simulink model "LoFT_Example1"  (R2022b)
settings: Solver=ode4  StartTime=0.0  StopTime=500  FixedStep=simu.dt  RelTol=1e-3
PreLoadFcn:
  | simu.dt = 0.0125;
  | simu.Tmax = 600;
undefined symbols (not defined in the file): body, circtime, Communication, irkb, LoFT, Turbwind, waves, wind
libraries: simulink x25
(part 1 of 4)
settings Model: SimulationMode=accelerator  Creator=85164  LastModifiedBy=85164

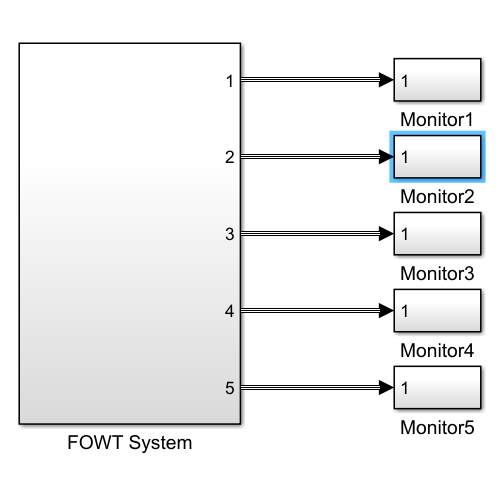
[thumbnail: Simulink's stored preview of the top-level diagram]
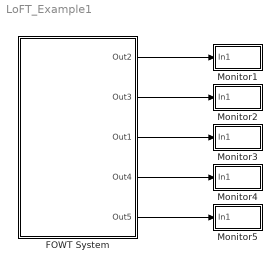
== system LoFT_Example1 ==
  FOWT System : Subsystem
  Monitor1 : Subsystem
  Monitor2 : Subsystem
  Monitor3 : Subsystem
  Monitor4 : Subsystem
  Monitor5 : Subsystem
  wires:
  FOWT System/1(Out2) -> Monitor1/1(In1)
  FOWT System/2(Out3) -> Monitor2/1(In1)
  FOWT System/3(Out1) -> Monitor3/1(In1)
  FOWT System/4(Out4) -> Monitor4/1(In1)
  FOWT System/5(Out5) -> Monitor5/1(In1)

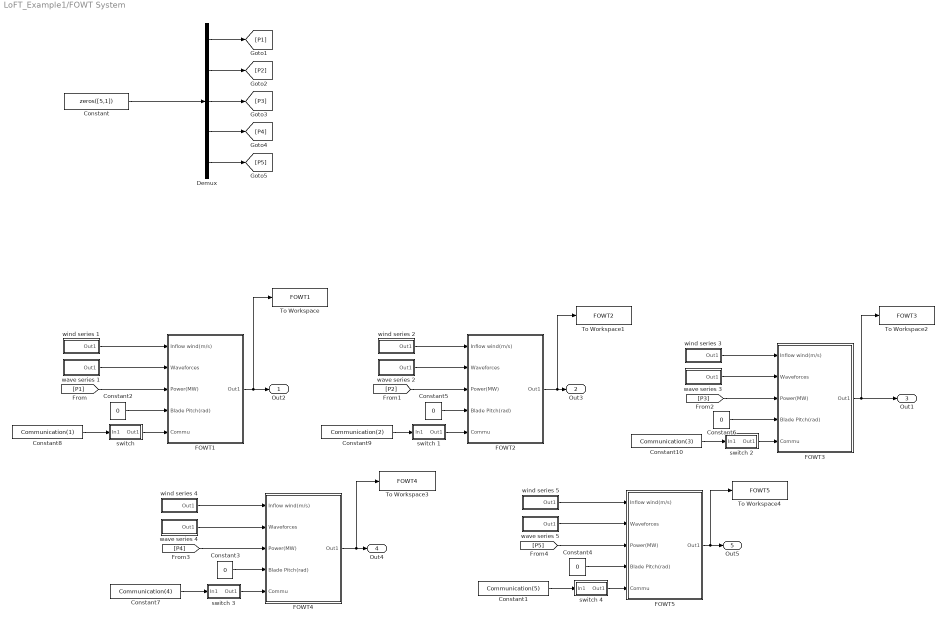
== system LoFT_Example1/FOWT System ==
  Constant : Constant  Value=zeros([5,1])
  Constant1 : Constant  Value=Communication(5)
  Constant10 : Constant  Value=Communication(3)
  Constant{2..6} (5 alike) : Constant  Value=0
  Constant7 : Constant  Value=Communication(4)
  Constant8 : Constant  Value=Communication(1)
  Constant9 : Constant  Value=Communication(2)
  Demux : Demux  Outputs=5
  FOWT1 : Subsystem  mask{Aero=LoFT.Aero, Hydro=LoFT.Hydro, Mooring=LoFT.Mooring, Property=LoFT.Property, Controller=LoFT.Controller, Initposition=[15,  0,  3*pi/180], Initstate=[6.8*pi/30, 9]}
      mask prompts: Aero "Aerodynamics"; Hydro "Hydrodynamics"; Mooring "Mooring lookup table"; Property "Hull mass, inertia and volume"; Controller "Local controller"; Initposition "Initial Hull position"; Initstate "Initial RotSpeed and WindEst"
      mask DialogControl DescGroupVar Prompt: LoFT
      mask DialogControl FOWT Prompt: Low-order modelling of floating offshore wind turbine for training
      mask DialogControl Manuscript Prompt: Citation
      mask DialogControl scriptname Prompt: Primary Frequency Response of Floating Offshore Wind Turbines via Deep Reinforcement Learning and Domain Randomization
      mask DialogControl ParameterGroupVar Prompt: 参数
  FOWT2 : Subsystem  mask{Aero=LoFT.Aero, Hydro=LoFT.Hydro, Mooring=LoFT.Mooring, Property=LoFT.Property, Controller=LoFT.Controller, Initposition=[15,  0,  3*pi/180], Initstate=[6.8*pi/30, 9]}
      mask prompts: Aero "Aerodynamics"; Hydro "Hydrodynamics"; Mooring "Mooring lookup table"; Property "Hull mass, inertia and volume"; Controller "Local controller"; Initposition "Initial Hull position"; Initstate "Initial RotSpeed and WindEst"
      mask DialogControl DescGroupVar Prompt: LoFT
      mask DialogControl FOWT Prompt: Low-order modelling of floating offshore wind turbine for training
      mask DialogControl Manuscript Prompt: Citation
      mask DialogControl scriptname Prompt: Primary Frequency Response of Floating Offshore Wind Turbines via Deep Reinforcement Learning and Domain Randomization
      mask DialogControl ParameterGroupVar Prompt: 参数
  FOWT3 : Subsystem  mask{Aero=LoFT.Aero, Hydro=LoFT.Hydro, Mooring=LoFT.Mooring, Property=LoFT.Property, Controller=LoFT.Controller, Initposition=[15,  0,  3*pi/180], Initstate=[6.8*pi/30, 9]}
      mask prompts: Aero "Aerodynamics"; Hydro "Hydrodynamics"; Mooring "Mooring lookup table"; Property "Hull mass, inertia and volume"; Controller "Local controller"; Initposition "Initial Hull position"; Initstate "Initial RotSpeed and WindEst"
      mask DialogControl DescGroupVar Prompt: LoFT
      mask DialogControl FOWT Prompt: Low-order modelling of floating offshore wind turbine for training
      mask DialogControl Manuscript Prompt: Citation
      mask DialogControl scriptname Prompt: Primary Frequency Response of Floating Offshore Wind Turbines via Deep Reinforcement Learning and Domain Randomization
      mask DialogControl ParameterGroupVar Prompt: 参数
  FOWT4 : Subsystem  mask{Aero=LoFT.Aero, Hydro=LoFT.Hydro, Mooring=LoFT.Mooring, Property=LoFT.Property, Controller=LoFT.Controller, Initposition=[15,  0,  3*pi/180], Initstate=[6.8*pi/30, 9]}
      mask prompts: Aero "Aerodynamics"; Hydro "Hydrodynamics"; Mooring "Mooring lookup table"; Property "Hull mass, inertia and volume"; Controller "Local controller"; Initposition "Initial Hull position"; Initstate "Initial RotSpeed and WindEst"
      mask DialogControl DescGroupVar Prompt: LoFT
      mask DialogControl FOWT Prompt: Low-order modelling of floating offshore wind turbine for training
      mask DialogControl Manuscript Prompt: Citation
      mask DialogControl scriptname Prompt: Primary Frequency Response of Floating Offshore Wind Turbines via Deep Reinforcement Learning and Domain Randomization
      mask DialogControl ParameterGroupVar Prompt: 参数
  FOWT5 : Subsystem  mask{Aero=LoFT.Aero, Hydro=LoFT.Hydro, Mooring=LoFT.Mooring, Property=LoFT.Property, Controller=LoFT.Controller, Initposition=[15,  0,  3*pi/180], Initstate=[6.8*pi/30, 9]}
      mask prompts: Aero "Aerodynamics"; Hydro "Hydrodynamics"; Mooring "Mooring lookup table"; Property "Hull mass, inertia and volume"; Controller "Local controller"; Initposition "Initial Hull position"; Initstate "Initial RotSpeed and WindEst"
      mask DialogControl DescGroupVar Prompt: LoFT
      mask DialogControl FOWT Prompt: Low-order modelling of floating offshore wind turbine for training
      mask DialogControl Manuscript Prompt: Citation
      mask DialogControl scriptname Prompt: Primary Frequency Response of Floating Offshore Wind Turbines via Deep Reinforcement Learning and Domain Randomization
      mask DialogControl ParameterGroupVar Prompt: 参数
  To Workspace : ToWorkspace  VariableName=FOWT1  SaveFormat=Timeseries  SampleTime=-1
  To Workspace1 : ToWorkspace  VariableName=FOWT2  SaveFormat=Timeseries  SampleTime=-1
  To Workspace2 : ToWorkspace  VariableName=FOWT3  SaveFormat=Timeseries  SampleTime=-1
  To Workspace3 : ToWorkspace  VariableName=FOWT4  SaveFormat=Timeseries  SampleTime=-1
  To Workspace4 : ToWorkspace  VariableName=FOWT5  SaveFormat=Timeseries  SampleTime=-1
  "switch " : Subsystem
  switch 1 : Subsystem
  switch 2 : Subsystem
  switch 3 : Subsystem
  switch 4 : Subsystem
  wave series 1 : Subsystem
  wave series 2 : Subsystem
  wave series 3 : Subsystem
  wave series 4 : Subsystem
  wave series 5 : Subsystem
  wind series 1 : Subsystem
  wind series 2 : Subsystem
  wind series 3 : Subsystem
  wind series 4 : Subsystem
  wind series 5 : Subsystem
  Out2 : Outport
  Out3 : Outport  Port=2
  Out1 : Outport  Port=3
  Out4 : Outport  Port=4
  Out5 : Outport  Port=5
  wires:
  switch 3/1(Out1) -> FOWT4/5(Commu)
  switch 4/1(Out1) -> FOWT5/5(Commu)
  wave series 4/1(Out1) -> FOWT4/2(Waveforces)
  switch 1/1(Out1) -> FOWT2/5(Commu)
  wave series 1/1(Out1) -> FOWT1/2(Waveforces)
  wave series 5/1(Out1) -> FOWT5/2(Waveforces)
  wave series 3/1(Out1) -> FOWT3/2(Waveforces)
  FOWT3/1(Out1) -> To Workspace2/1, Out1/1
  wave series 2/1(Out1) -> FOWT2/2(Waveforces)
  "switch "/1(Out1) -> FOWT1/5(Commu)
  switch 2/1(Out1) -> FOWT3/5(Commu)
  [P1] -> FOWT1/3(Power(MW))
  Constant2/1 -> FOWT1/4(Blade Pitch(rad))
  FOWT4/1(Out1) -> To Workspace3/1, Out4/1
  FOWT5/1(Out1) -> To Workspace4/1, Out5/1
  Constant1/1 -> switch 4/1(In1)
  [P2] -> FOWT2/3(Power(MW))
  [P3] -> FOWT3/3(Power(MW))
  Constant3/1 -> FOWT4/4(Blade Pitch(rad))
  Constant4/1 -> FOWT5/4(Blade Pitch(rad))
  Constant5/1 -> FOWT2/4(Blade Pitch(rad))
  Constant6/1 -> FOWT3/4(Blade Pitch(rad))
  Demux/1 -> [P1]
  Demux/5 -> [P5]
  Demux/4 -> [P4]
  Demux/3 -> [P3]
  Demux/2 -> [P2]
  [P4] -> FOWT4/3(Power(MW))
  [P5] -> FOWT5/3(Power(MW))
  FOWT2/1(Out1) -> To Workspace1/1, Out3/1
  Constant7/1 -> switch 3/1(In1)
  Constant8/1 -> "switch "/1(In1)
  Constant9/1 -> switch 1/1(In1)
  Constant10/1 -> switch 2/1(In1)
  Constant/1 -> Demux/1
  FOWT1/1(Out1) -> To Workspace/1, Out2/1
  wind series 5/1(Out1) -> FOWT5/1(Inflow wind(m/s))
  wind series 4/1(Out1) -> FOWT4/1(Inflow wind(m/s))
  wind series 3/1(Out1) -> FOWT3/1(Inflow wind(m/s))
  wind series 1/1(Out1) -> FOWT1/1(Inflow wind(m/s))
  wind series 2/1(Out1) -> FOWT2/1(Inflow wind(m/s))

== system LoFT_Example1/Monitor1 ==
  In1 : Inport
  Bus Selector : BusSelector  OutputSignals=PtfmSurge,PtfmHeave,PtfmPitch,WindVelX,WindEst,BldPitch,RotSpeed,GenPwr,RotThrust,GenTorq,RotTorq
  Gain : Gain  Gain=180/pi
  Gain1 : Gain  Gain=180/pi
  Scope : Scope  NumInputPorts=11
      settings: StartFcn=open_system(gcbh)
  wires:
  In1/1 -> Bus Selector/1
  Bus Selector/1 -> Scope/1  "<PtfmSurge>"
  Bus Selector/2 -> Scope/2  "<PtfmHeave>"
  Bus Selector/4 -> Scope/4  "<WindVelX>"
  Bus Selector/5 -> Scope/5  "<WindEst>"
  Bus Selector/7 -> Scope/7  "<RotSpeed>"
  Bus Selector/8 -> Scope/8  "<GenPwr>"
  Bus Selector/9 -> Scope/9  "<RotThrust>"
  Bus Selector/10 -> Scope/10  "<GenTorq>"
  Bus Selector/3 -> Gain/1  "<PtfmPitch>"
  Gain/1 -> Scope/3  "PtfmPitch"
  Bus Selector/6 -> Gain1/1  "<BldPitch>"
  Gain1/1 -> Scope/6  "BldPitch"
  Bus Selector/11 -> Scope/11  "<RotTorq>"

== system LoFT_Example1/Monitor2 ==
  In1 : Inport
  Bus Selector : BusSelector  OutputSignals=PtfmSurge,PtfmHeave,PtfmPitch,WindVelX,WindEst,BldPitch,RotSpeed,GenPwr,RotThrust,GenTorq,RotTorq
  Gain : Gain  Gain=180/pi
  Gain1 : Gain  Gain=180/pi
  Scope : Scope  NumInputPorts=11
  wires:
  Bus Selector/11 -> Scope/11  "<RotTorq>"
  Gain1/1 -> Scope/6  "BldPitch"
  Bus Selector/6 -> Gain1/1  "<BldPitch>"
  Gain/1 -> Scope/3  "PtfmPitch"
  Bus Selector/3 -> Gain/1  "<PtfmPitch>"
  Bus Selector/10 -> Scope/10  "<GenTorq>"
  Bus Selector/9 -> Scope/9  "<RotThrust>"
  Bus Selector/8 -> Scope/8  "<GenPwr>"
  Bus Selector/7 -> Scope/7  "<RotSpeed>"
  Bus Selector/5 -> Scope/5  "<WindEst>"
  Bus Selector/4 -> Scope/4  "<WindVelX>"
  Bus Selector/2 -> Scope/2  "<PtfmHeave>"
  Bus Selector/1 -> Scope/1  "<PtfmSurge>"
  In1/1 -> Bus Selector/1

== system LoFT_Example1/Monitor3 ==
  In1 : Inport
  Bus Selector : BusSelector  OutputSignals=PtfmSurge,PtfmHeave,PtfmPitch,WindVelX,WindEst,BldPitch,RotSpeed,GenPwr,RotThrust,GenTorq,RotTorq
  Gain : Gain  Gain=180/pi
  Gain1 : Gain  Gain=180/pi
  Scope : Scope  NumInputPorts=11
  wires:
  In1/1 -> Bus Selector/1
  Bus Selector/1 -> Scope/1  "<PtfmSurge>"
  Bus Selector/2 -> Scope/2  "<PtfmHeave>"
  Bus Selector/4 -> Scope/4  "<WindVelX>"
  Bus Selector/5 -> Scope/5  "<WindEst>"
  Bus Selector/7 -> Scope/7  "<RotSpeed>"
  Bus Selector/8 -> Scope/8  "<GenPwr>"
  Bus Selector/9 -> Scope/9  "<RotThrust>"
  Bus Selector/10 -> Scope/10  "<GenTorq>"
  Bus Selector/3 -> Gain/1  "<PtfmPitch>"
  Gain/1 -> Scope/3  "PtfmPitch"
  Bus Selector/6 -> Gain1/1  "<BldPitch>"
  Gain1/1 -> Scope/6  "BldPitch"
  Bus Selector/11 -> Scope/11  "<RotTorq>"

== system LoFT_Example1/Monitor4 ==
  In1 : Inport
  Bus Selector : BusSelector  OutputSignals=PtfmSurge,PtfmHeave,PtfmPitch,WindVelX,WindEst,BldPitch,RotSpeed,GenPwr,RotThrust,GenTorq,RotTorq
  Gain : Gain  Gain=180/pi
  Gain1 : Gain  Gain=180/pi
  Scope : Scope  NumInputPorts=11
  wires:
  Bus Selector/11 -> Scope/11  "<RotTorq>"
  Gain1/1 -> Scope/6  "BldPitch"
  Bus Selector/6 -> Gain1/1  "<BldPitch>"
  Gain/1 -> Scope/3  "PtfmPitch"
  Bus Selector/3 -> Gain/1  "<PtfmPitch>"
  Bus Selector/10 -> Scope/10  "<GenTorq>"
  Bus Selector/9 -> Scope/9  "<RotThrust>"
  Bus Selector/8 -> Scope/8  "<GenPwr>"
  Bus Selector/7 -> Scope/7  "<RotSpeed>"
  Bus Selector/5 -> Scope/5  "<WindEst>"
  Bus Selector/4 -> Scope/4  "<WindVelX>"
  Bus Selector/2 -> Scope/2  "<PtfmHeave>"
  Bus Selector/1 -> Scope/1  "<PtfmSurge>"
  In1/1 -> Bus Selector/1

== system LoFT_Example1/Monitor5 ==
  In1 : Inport
  Bus Selector : BusSelector  OutputSignals=PtfmSurge,PtfmHeave,PtfmPitch,WindVelX,WindEst,BldPitch,RotSpeed,GenPwr,RotThrust,GenTorq,RotTorq
  Gain : Gain  Gain=180/pi
  Gain1 : Gain  Gain=180/pi
  Scope : Scope  NumInputPorts=11
  wires:
  In1/1 -> Bus Selector/1
  Bus Selector/1 -> Scope/1  "<PtfmSurge>"
  Bus Selector/2 -> Scope/2  "<PtfmHeave>"
  Bus Selector/4 -> Scope/4  "<WindVelX>"
  Bus Selector/5 -> Scope/5  "<WindEst>"
  Bus Selector/7 -> Scope/7  "<RotSpeed>"
  Bus Selector/8 -> Scope/8  "<GenPwr>"
  Bus Selector/9 -> Scope/9  "<RotThrust>"
  Bus Selector/10 -> Scope/10  "<GenTorq>"
  Bus Selector/3 -> Gain/1  "<PtfmPitch>"
  Gain/1 -> Scope/3  "PtfmPitch"
  Bus Selector/6 -> Gain1/1  "<BldPitch>"
  Gain1/1 -> Scope/6  "BldPitch"
  Bus Selector/11 -> Scope/11  "<RotTorq>"

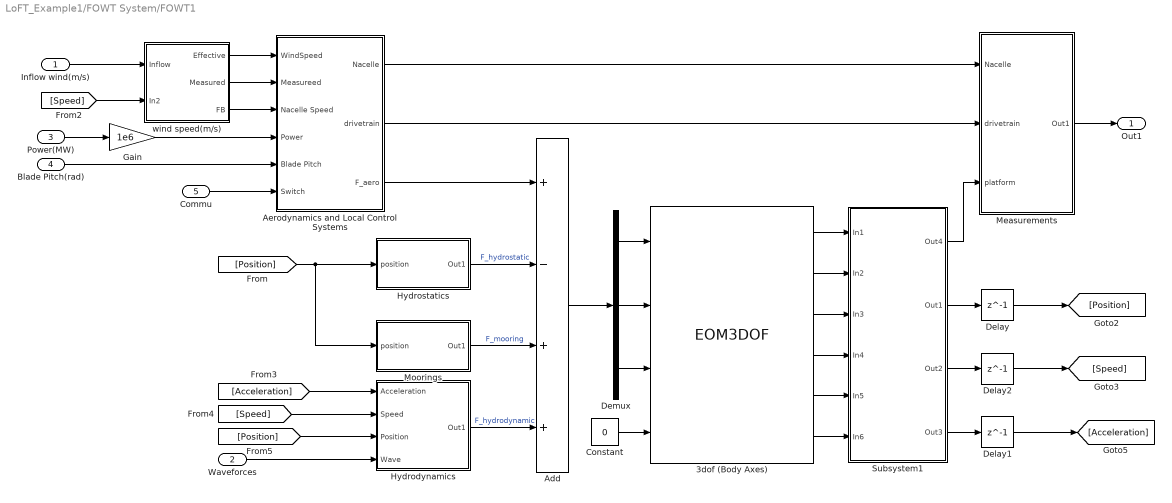
== system LoFT_Example1/FOWT System/FOWT1 ==
  Inflow wind(m/s) : Inport
  Waveforces : Inport  Port=2
  Power(MW) : Inport  Port=3
  Blade Pitch(rad) : Inport  Port=4
  Commu : Inport  Port=5
  3dof (Body Axes) : EOM3DOF  v_ini=0.01  theta_ini=Initposition(3)  pos_ini=[Initposition(1) Initposition(2)]  mass=Property.masstot  Iyy=Property.pitchinertia  g_in=External
  Add : Sum  Inputs=+-++
  Aerodynamics and Local Control Systems : Subsystem
  Constant : Constant  Value=0
  Delay : Delay  DelayLength=1  InitialCondition=0
  Delay1 : Delay  DelayLength=1  InitialCondition=0
  Delay2 : Delay  DelayLength=1  InitialCondition=0
  Demux : Demux  Outputs=3
  Gain : Gain  Gain=1e6
  Hydrodynamics : Subsystem
  Hydrostatics : Subsystem
  Measurements : Subsystem
  Moorings : Subsystem
  Subsystem1 : Subsystem
  wind speed(m/s) : Subsystem
  Out1 : Outport
  wires:
  Power(MW)/1 -> Gain/1
  wind speed(m/s)/3(FB) -> Aerodynamics and Local Control Systems/3(Nacelle Speed)
  Aerodynamics and Local Control Systems/2(drivetrain) -> Measurements/2(drivetrain)
  Measurements/1(Out1) -> Out1/1
  Aerodynamics and Local Control Systems/1(Nacelle) -> Measurements/1(Nacelle)
  Subsystem1/1(Out4) -> Measurements/3(platform)
  Waveforces/1 -> Hydrodynamics/4(Wave)
  Commu/1 -> Aerodynamics and Local Control Systems/6(Switch)
  Aerodynamics and Local Control Systems/3(F_aero) -> Add/1
  [Speed] -> wind speed(m/s)/2(In2)
  [Position] -> Hydrodynamics/3(Position)
  Hydrodynamics/1(Out1) -> Add/4  "F_hydrodynamic"
  [Speed] -> Hydrodynamics/2(Speed)
  Demux/3 -> 3dof (Body Axes)/3
  Demux/2 -> 3dof (Body Axes)/2
  Demux/1 -> 3dof (Body Axes)/1
  Add/1 -> Demux/1
  3dof (Body Axes)/6 -> Subsystem1/6(In6)
  3dof (Body Axes)/5 -> Subsystem1/5(In5)
  3dof (Body Axes)/4 -> Subsystem1/4(In4)
  3dof (Body Axes)/3 -> Subsystem1/3(In3)
  3dof (Body Axes)/2 -> Subsystem1/2(In2)
  3dof (Body Axes)/1 -> Subsystem1/1(In1)
  Moorings/1(Out1) -> Add/3  "F_mooring"
  Constant/1 -> 3dof (Body Axes)/4
  Hydrostatics/1(Out1) -> Add/2  "F_hydrostatic"
  [Position] -> Hydrostatics/1(position), Moorings/1(position)
  wind speed(m/s)/1(Effective) -> Aerodynamics and Local Control Systems/1(WindSpeed)
  Subsystem1/2(Out1) -> Delay/1
  Gain/1 -> Aerodynamics and Local Control Systems/4(Power)
  Subsystem1/3(Out2) -> Delay2/1
  Subsystem1/4(Out3) -> Delay1/1
  Inflow wind(m/s)/1 -> wind speed(m/s)/1(Inflow)
  Delay1/1 -> [Acceleration]
  Delay2/1 -> [Speed]
  Delay/1 -> [Position]
  [Acceleration] -> Hydrodynamics/1(Acceleration)
  wind speed(m/s)/2(Measured) -> Aerodynamics and Local Control Systems/2("Measureed ")
  Blade Pitch(rad)/1 -> Aerodynamics and Local Control Systems/5(Blade Pitch)

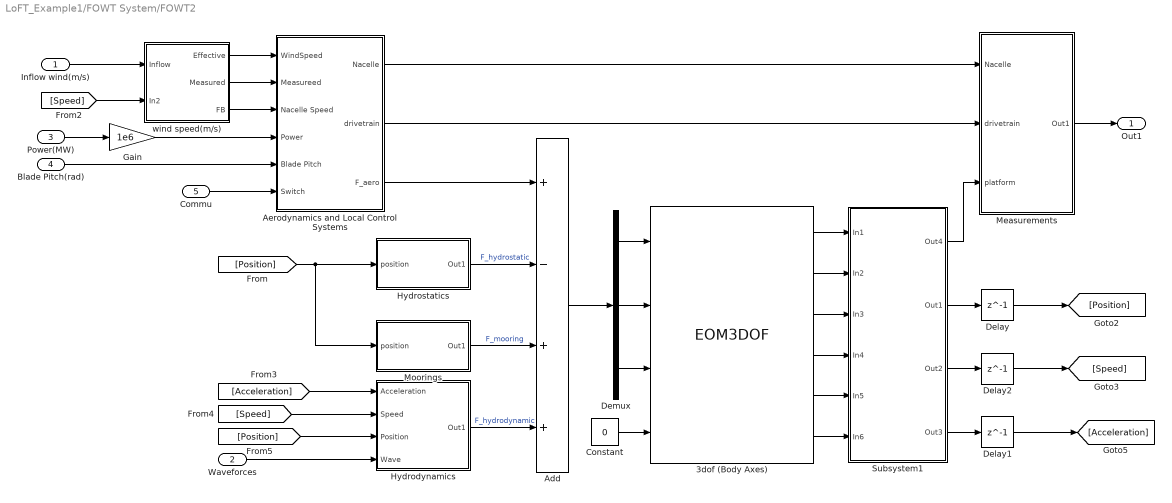
== system LoFT_Example1/FOWT System/FOWT2 ==
  Inflow wind(m/s) : Inport
  Waveforces : Inport  Port=2
  Power(MW) : Inport  Port=3
  Blade Pitch(rad) : Inport  Port=4
  Commu : Inport  Port=5
  3dof (Body Axes) : EOM3DOF  v_ini=0.01  theta_ini=Initposition(3)  pos_ini=[Initposition(1) Initposition(2)]  mass=Property.masstot  Iyy=Property.pitchinertia  g_in=External
  Add : Sum  Inputs=+-++
  Aerodynamics and Local Control Systems : Subsystem
  Constant : Constant  Value=0
  Delay : Delay  DelayLength=1  InitialCondition=0
  Delay1 : Delay  DelayLength=1  InitialCondition=0
  Delay2 : Delay  DelayLength=1  InitialCondition=0
  Demux : Demux  Outputs=3
  Gain : Gain  Gain=1e6
  Hydrodynamics : Subsystem
  Hydrostatics : Subsystem
  Measurements : Subsystem
  Moorings : Subsystem
  Subsystem1 : Subsystem
  wind speed(m/s) : Subsystem
  Out1 : Outport
  wires:
  Blade Pitch(rad)/1 -> Aerodynamics and Local Control Systems/5(Blade Pitch)
  wind speed(m/s)/2(Measured) -> Aerodynamics and Local Control Systems/2("Measureed ")
  [Acceleration] -> Hydrodynamics/1(Acceleration)
  Delay/1 -> [Position]
  Delay2/1 -> [Speed]
  Delay1/1 -> [Acceleration]
  Inflow wind(m/s)/1 -> wind speed(m/s)/1(Inflow)
  Subsystem1/4(Out3) -> Delay1/1
  Subsystem1/3(Out2) -> Delay2/1
  Gain/1 -> Aerodynamics and Local Control Systems/4(Power)
  Subsystem1/2(Out1) -> Delay/1
  wind speed(m/s)/1(Effective) -> Aerodynamics and Local Control Systems/1(WindSpeed)
  [Position] -> Moorings/1(position), Hydrostatics/1(position)
  Hydrostatics/1(Out1) -> Add/2  "F_hydrostatic"
  Constant/1 -> 3dof (Body Axes)/4
  Moorings/1(Out1) -> Add/3  "F_mooring"
  3dof (Body Axes)/1 -> Subsystem1/1(In1)
  3dof (Body Axes)/2 -> Subsystem1/2(In2)
  3dof (Body Axes)/3 -> Subsystem1/3(In3)
  3dof (Body Axes)/4 -> Subsystem1/4(In4)
  3dof (Body Axes)/5 -> Subsystem1/5(In5)
  3dof (Body Axes)/6 -> Subsystem1/6(In6)
  Add/1 -> Demux/1
  Demux/1 -> 3dof (Body Axes)/1
  Demux/2 -> 3dof (Body Axes)/2
  Demux/3 -> 3dof (Body Axes)/3
  [Speed] -> Hydrodynamics/2(Speed)
  Hydrodynamics/1(Out1) -> Add/4  "F_hydrodynamic"
  [Position] -> Hydrodynamics/3(Position)
  [Speed] -> wind speed(m/s)/2(In2)
  Aerodynamics and Local Control Systems/3(F_aero) -> Add/1
  Commu/1 -> Aerodynamics and Local Control Systems/6(Switch)
  Waveforces/1 -> Hydrodynamics/4(Wave)
  Subsystem1/1(Out4) -> Measurements/3(platform)
  Aerodynamics and Local Control Systems/1(Nacelle) -> Measurements/1(Nacelle)
  Measurements/1(Out1) -> Out1/1
  Aerodynamics and Local Control Systems/2(drivetrain) -> Measurements/2(drivetrain)
  wind speed(m/s)/3(FB) -> Aerodynamics and Local Control Systems/3(Nacelle Speed)
  Power(MW)/1 -> Gain/1

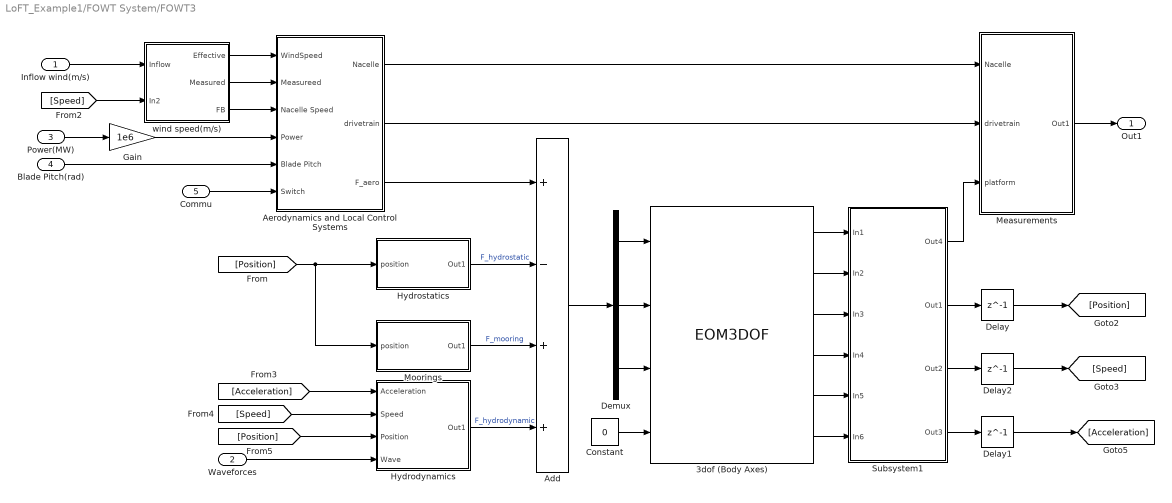
== system LoFT_Example1/FOWT System/FOWT3 ==
  Inflow wind(m/s) : Inport
  Waveforces : Inport  Port=2
  Power(MW) : Inport  Port=3
  Blade Pitch(rad) : Inport  Port=4
  Commu : Inport  Port=5
  3dof (Body Axes) : EOM3DOF  v_ini=0.01  theta_ini=Initposition(3)  pos_ini=[Initposition(1) Initposition(2)]  mass=Property.masstot  Iyy=Property.pitchinertia  g_in=External
  Add : Sum  Inputs=+-++
  Aerodynamics and Local Control Systems : Subsystem
  Constant : Constant  Value=0
  Delay : Delay  DelayLength=1  InitialCondition=0
  Delay1 : Delay  DelayLength=1  InitialCondition=0
  Delay2 : Delay  DelayLength=1  InitialCondition=0
  Demux : Demux  Outputs=3
  Gain : Gain  Gain=1e6
  Hydrodynamics : Subsystem
  Hydrostatics : Subsystem
  Measurements : Subsystem
  Moorings : Subsystem
  Subsystem1 : Subsystem
  wind speed(m/s) : Subsystem
  Out1 : Outport
  wires:
  Power(MW)/1 -> Gain/1
  wind speed(m/s)/3(FB) -> Aerodynamics and Local Control Systems/3(Nacelle Speed)
  Aerodynamics and Local Control Systems/2(drivetrain) -> Measurements/2(drivetrain)
  Measurements/1(Out1) -> Out1/1
  Aerodynamics and Local Control Systems/1(Nacelle) -> Measurements/1(Nacelle)
  Subsystem1/1(Out4) -> Measurements/3(platform)
  Waveforces/1 -> Hydrodynamics/4(Wave)
  Commu/1 -> Aerodynamics and Local Control Systems/6(Switch)
  Aerodynamics and Local Control Systems/3(F_aero) -> Add/1
  [Speed] -> wind speed(m/s)/2(In2)
  [Position] -> Hydrodynamics/3(Position)
  Hydrodynamics/1(Out1) -> Add/4  "F_hydrodynamic"
  [Speed] -> Hydrodynamics/2(Speed)
  Demux/3 -> 3dof (Body Axes)/3
  Demux/2 -> 3dof (Body Axes)/2
  Demux/1 -> 3dof (Body Axes)/1
  Add/1 -> Demux/1
  3dof (Body Axes)/6 -> Subsystem1/6(In6)
  3dof (Body Axes)/5 -> Subsystem1/5(In5)
  3dof (Body Axes)/4 -> Subsystem1/4(In4)
  3dof (Body Axes)/3 -> Subsystem1/3(In3)
  3dof (Body Axes)/2 -> Subsystem1/2(In2)
  3dof (Body Axes)/1 -> Subsystem1/1(In1)
  Moorings/1(Out1) -> Add/3  "F_mooring"
  Constant/1 -> 3dof (Body Axes)/4
  Hydrostatics/1(Out1) -> Add/2  "F_hydrostatic"
  [Position] -> Hydrostatics/1(position), Moorings/1(position)
  wind speed(m/s)/1(Effective) -> Aerodynamics and Local Control Systems/1(WindSpeed)
  Subsystem1/2(Out1) -> Delay/1
  Gain/1 -> Aerodynamics and Local Control Systems/4(Power)
  Subsystem1/3(Out2) -> Delay2/1
  Subsystem1/4(Out3) -> Delay1/1
  Inflow wind(m/s)/1 -> wind speed(m/s)/1(Inflow)
  Delay1/1 -> [Acceleration]
  Delay2/1 -> [Speed]
  Delay/1 -> [Position]
  [Acceleration] -> Hydrodynamics/1(Acceleration)
  wind speed(m/s)/2(Measured) -> Aerodynamics and Local Control Systems/2("Measureed ")
  Blade Pitch(rad)/1 -> Aerodynamics and Local Control Systems/5(Blade Pitch)

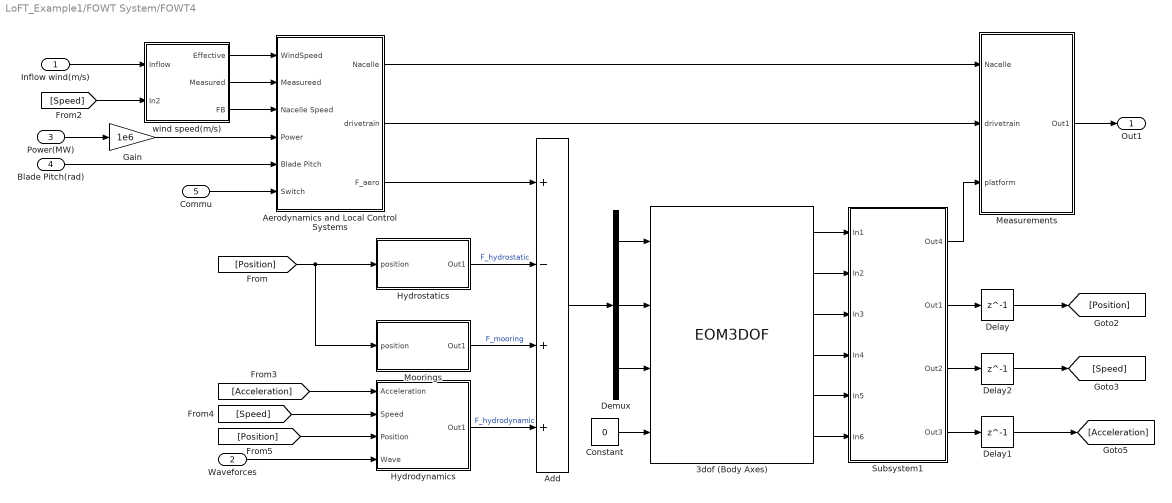
== system LoFT_Example1/FOWT System/FOWT4 ==
  Inflow wind(m/s) : Inport
  Waveforces : Inport  Port=2
  Power(MW) : Inport  Port=3
  Blade Pitch(rad) : Inport  Port=4
  Commu : Inport  Port=5
  3dof (Body Axes) : EOM3DOF  v_ini=0.01  theta_ini=Initposition(3)  pos_ini=[Initposition(1) Initposition(2)]  mass=Property.masstot  Iyy=Property.pitchinertia  g_in=External
  Add : Sum  Inputs=+-++
  Aerodynamics and Local Control Systems : Subsystem
  Constant : Constant  Value=0
  Delay : Delay  DelayLength=1  InitialCondition=0
  Delay1 : Delay  DelayLength=1  InitialCondition=0
  Delay2 : Delay  DelayLength=1  InitialCondition=0
  Demux : Demux  Outputs=3
  Gain : Gain  Gain=1e6
  Hydrodynamics : Subsystem
  Hydrostatics : Subsystem
  Measurements : Subsystem
  Moorings : Subsystem
  Subsystem1 : Subsystem
  wind speed(m/s) : Subsystem
  Out1 : Outport
  wires:
  Blade Pitch(rad)/1 -> Aerodynamics and Local Control Systems/5(Blade Pitch)
  wind speed(m/s)/2(Measured) -> Aerodynamics and Local Control Systems/2("Measureed ")
  [Acceleration] -> Hydrodynamics/1(Acceleration)
  Delay/1 -> [Position]
  Delay2/1 -> [Speed]
  Delay1/1 -> [Acceleration]
  Inflow wind(m/s)/1 -> wind speed(m/s)/1(Inflow)
  Subsystem1/4(Out3) -> Delay1/1
  Subsystem1/3(Out2) -> Delay2/1
  Gain/1 -> Aerodynamics and Local Control Systems/4(Power)
  Subsystem1/2(Out1) -> Delay/1
  wind speed(m/s)/1(Effective) -> Aerodynamics and Local Control Systems/1(WindSpeed)
  [Position] -> Moorings/1(position), Hydrostatics/1(position)
  Hydrostatics/1(Out1) -> Add/2  "F_hydrostatic"
  Constant/1 -> 3dof (Body Axes)/4
  Moorings/1(Out1) -> Add/3  "F_mooring"
  3dof (Body Axes)/1 -> Subsystem1/1(In1)
  3dof (Body Axes)/2 -> Subsystem1/2(In2)
  3dof (Body Axes)/3 -> Subsystem1/3(In3)
  3dof (Body Axes)/4 -> Subsystem1/4(In4)
  3dof (Body Axes)/5 -> Subsystem1/5(In5)
  3dof (Body Axes)/6 -> Subsystem1/6(In6)
  Add/1 -> Demux/1
  Demux/1 -> 3dof (Body Axes)/1
  Demux/2 -> 3dof (Body Axes)/2
  Demux/3 -> 3dof (Body Axes)/3
  [Speed] -> Hydrodynamics/2(Speed)
  Hydrodynamics/1(Out1) -> Add/4  "F_hydrodynamic"
  [Position] -> Hydrodynamics/3(Position)
  [Speed] -> wind speed(m/s)/2(In2)
  Aerodynamics and Local Control Systems/3(F_aero) -> Add/1
  Commu/1 -> Aerodynamics and Local Control Systems/6(Switch)
  Waveforces/1 -> Hydrodynamics/4(Wave)
  Subsystem1/1(Out4) -> Measurements/3(platform)
  Aerodynamics and Local Control Systems/1(Nacelle) -> Measurements/1(Nacelle)
  Measurements/1(Out1) -> Out1/1
  Aerodynamics and Local Control Systems/2(drivetrain) -> Measurements/2(drivetrain)
  wind speed(m/s)/3(FB) -> Aerodynamics and Local Control Systems/3(Nacelle Speed)
  Power(MW)/1 -> Gain/1

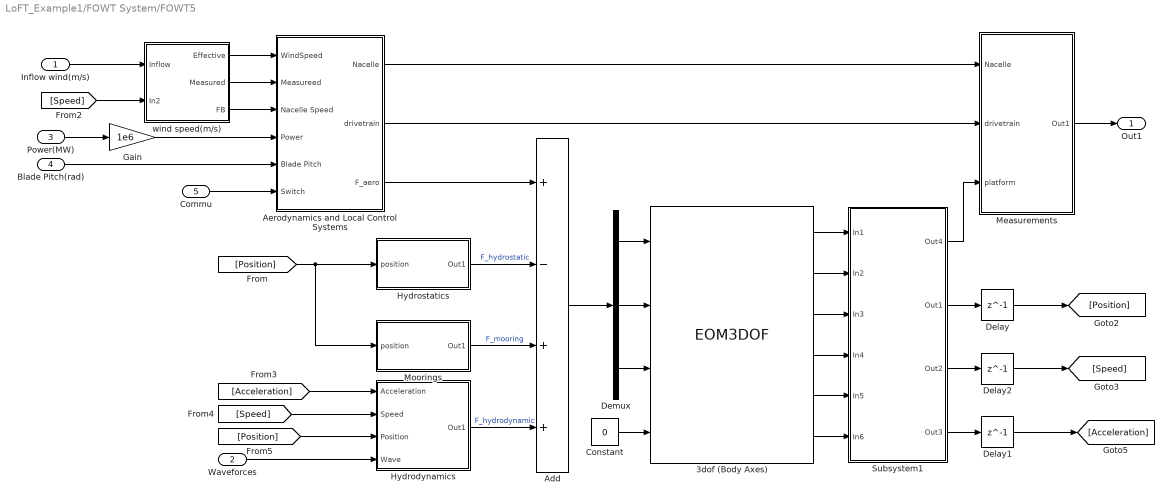
== system LoFT_Example1/FOWT System/FOWT5 ==
  Inflow wind(m/s) : Inport
  Waveforces : Inport  Port=2
  Power(MW) : Inport  Port=3
  Blade Pitch(rad) : Inport  Port=4
  Commu : Inport  Port=5
  3dof (Body Axes) : EOM3DOF  v_ini=0.01  theta_ini=Initposition(3)  pos_ini=[Initposition(1) Initposition(2)]  mass=Property.masstot  Iyy=Property.pitchinertia  g_in=External
  Add : Sum  Inputs=+-++
  Aerodynamics and Local Control Systems : Subsystem
  Constant : Constant  Value=0
  Delay : Delay  DelayLength=1  InitialCondition=0
  Delay1 : Delay  DelayLength=1  InitialCondition=0
  Delay2 : Delay  DelayLength=1  InitialCondition=0
  Demux : Demux  Outputs=3
  Gain : Gain  Gain=1e6
  Hydrodynamics : Subsystem
  Hydrostatics : Subsystem
  Measurements : Subsystem
  Moorings : Subsystem
  Subsystem1 : Subsystem
  wind speed(m/s) : Subsystem
  Out1 : Outport
  wires:
  Power(MW)/1 -> Gain/1
  wind speed(m/s)/3(FB) -> Aerodynamics and Local Control Systems/3(Nacelle Speed)
  Aerodynamics and Local Control Systems/2(drivetrain) -> Measurements/2(drivetrain)
  Measurements/1(Out1) -> Out1/1
  Aerodynamics and Local Control Systems/1(Nacelle) -> Measurements/1(Nacelle)
  Subsystem1/1(Out4) -> Measurements/3(platform)
  Waveforces/1 -> Hydrodynamics/4(Wave)
  Commu/1 -> Aerodynamics and Local Control Systems/6(Switch)
  Aerodynamics and Local Control Systems/3(F_aero) -> Add/1
  [Speed] -> wind speed(m/s)/2(In2)
  [Position] -> Hydrodynamics/3(Position)
  Hydrodynamics/1(Out1) -> Add/4  "F_hydrodynamic"
  [Speed] -> Hydrodynamics/2(Speed)
  Demux/3 -> 3dof (Body Axes)/3
  Demux/2 -> 3dof (Body Axes)/2
  Demux/1 -> 3dof (Body Axes)/1
  Add/1 -> Demux/1
  3dof (Body Axes)/6 -> Subsystem1/6(In6)
  3dof (Body Axes)/5 -> Subsystem1/5(In5)
  3dof (Body Axes)/4 -> Subsystem1/4(In4)
  3dof (Body Axes)/3 -> Subsystem1/3(In3)
  3dof (Body Axes)/2 -> Subsystem1/2(In2)
  3dof (Body Axes)/1 -> Subsystem1/1(In1)
  Moorings/1(Out1) -> Add/3  "F_mooring"
  Constant/1 -> 3dof (Body Axes)/4
  Hydrostatics/1(Out1) -> Add/2  "F_hydrostatic"
  [Position] -> Hydrostatics/1(position), Moorings/1(position)
  wind speed(m/s)/1(Effective) -> Aerodynamics and Local Control Systems/1(WindSpeed)
  Subsystem1/2(Out1) -> Delay/1
  Gain/1 -> Aerodynamics and Local Control Systems/4(Power)
  Subsystem1/3(Out2) -> Delay2/1
  Subsystem1/4(Out3) -> Delay1/1
  Inflow wind(m/s)/1 -> wind speed(m/s)/1(Inflow)
  Delay1/1 -> [Acceleration]
  Delay2/1 -> [Speed]
  Delay/1 -> [Position]
  [Acceleration] -> Hydrodynamics/1(Acceleration)
  wind speed(m/s)/2(Measured) -> Aerodynamics and Local Control Systems/2("Measureed ")
  Blade Pitch(rad)/1 -> Aerodynamics and Local Control Systems/5(Blade Pitch)

== system LoFT_Example1/FOWT System/switch  ==
  note: communictation failure occurs when switch ==0
  In1 : Inport
  Constant : Constant  Value=0
  Mux : Mux  Inputs=2
  Out1 : Outport
  wires:
  Mux/1 -> Out1/1
  In1/1 -> Mux/1
  Constant/1 -> Mux/2

== system LoFT_Example1/FOWT System/switch 1 ==
  note: communictation failure occurs when switch ==0
  In1 : Inport
  Constant : Constant  Value=0
  Mux : Mux  Inputs=2
  Out1 : Outport
  wires:
  Constant/1 -> Mux/2
  In1/1 -> Mux/1
  Mux/1 -> Out1/1

== system LoFT_Example1/FOWT System/switch 2 ==
  note: communictation failure occurs when switch ==0
  In1 : Inport
  Constant : Constant  Value=0
  Mux : Mux  Inputs=2
  Out1 : Outport
  wires:
  Mux/1 -> Out1/1
  In1/1 -> Mux/1
  Constant/1 -> Mux/2

== system LoFT_Example1/FOWT System/switch 3 ==
  note: communictation failure occurs when switch ==0
  In1 : Inport
  Constant : Constant  Value=0
  Mux : Mux  Inputs=2
  Out1 : Outport
  wires:
  Constant/1 -> Mux/2
  In1/1 -> Mux/1
  Mux/1 -> Out1/1

== system LoFT_Example1/FOWT System/switch 4 ==
  note: communictation failure occurs when switch ==0
  In1 : Inport
  Constant : Constant  Value=0
  Mux : Mux  Inputs=2
  Out1 : Outport
  wires:
  Mux/1 -> Out1/1
  In1/1 -> Mux/1
  Constant/1 -> Mux/2

== system LoFT_Example1/FOWT System/wave series 1 ==
  1-D Lookup Table : Lookup_n-D  NumberOfTableDimensions=1  BreakpointsForDimension1=LoFT.Hydro.waveforces.time  Table=squeeze(LoFT.Hydro.waveforces.force(1,1,:))  InternalRulePriority=Speed  RndMeth=Simplest
  1-D Lookup Table1 : Lookup_n-D  NumberOfTableDimensions=1  BreakpointsForDimension1=LoFT.Hydro.waveforces.time  Table=squeeze(LoFT.Hydro.waveforces.force(1,2,:))  InternalRulePriority=Speed  RndMeth=Simplest
  1-D Lookup Table2 : Lookup_n-D  NumberOfTableDimensions=1  BreakpointsForDimension1=LoFT.Hydro.waveforces.time  Table=squeeze(LoFT.Hydro.waveforces.force(1,3,:))  InternalRulePriority=Speed  RndMeth=Simplest
  Clock1 : Clock
  Clock2 : Clock
  Clock3 : Clock
  Vector Concatenate1 : Concatenate  NumInputs=3
  Out1 : Outport
  wires:
  Vector Concatenate1/1 -> Out1/1
  Clock2/1 -> 1-D Lookup Table1/1
  1-D Lookup Table/1 -> Vector Concatenate1/1
  Clock3/1 -> 1-D Lookup Table2/1
  Clock1/1 -> 1-D Lookup Table/1
  1-D Lookup Table1/1 -> Vector Concatenate1/2
  1-D Lookup Table2/1 -> Vector Concatenate1/3

== system LoFT_Example1/FOWT System/wave series 2 ==
  1-D Lookup Table : Lookup_n-D  NumberOfTableDimensions=1  BreakpointsForDimension1=LoFT.Hydro.waveforces.time + 5  Table=squeeze(LoFT.Hydro.waveforces.force(1,1,:))  InternalRulePriority=Speed  RndMeth=Simplest
  1-D Lookup Table1 : Lookup_n-D  NumberOfTableDimensions=1  BreakpointsForDimension1=LoFT.Hydro.waveforces.time + 5  Table=squeeze(LoFT.Hydro.waveforces.force(1,2,:))  InternalRulePriority=Speed  RndMeth=Simplest
  1-D Lookup Table2 : Lookup_n-D  NumberOfTableDimensions=1  BreakpointsForDimension1=LoFT.Hydro.waveforces.time + 5  Table=squeeze(LoFT.Hydro.waveforces.force(1,3,:))  InternalRulePriority=Speed  RndMeth=Simplest
  Clock1 : Clock
  Clock2 : Clock
  Clock3 : Clock
  Vector Concatenate1 : Concatenate  NumInputs=3
  Out1 : Outport
  wires:
  1-D Lookup Table2/1 -> Vector Concatenate1/3
  1-D Lookup Table1/1 -> Vector Concatenate1/2
  Clock1/1 -> 1-D Lookup Table/1
  Clock3/1 -> 1-D Lookup Table2/1
  1-D Lookup Table/1 -> Vector Concatenate1/1
  Clock2/1 -> 1-D Lookup Table1/1
  Vector Concatenate1/1 -> Out1/1

== system LoFT_Example1/FOWT System/wave series 3 ==
  1-D Lookup Table : Lookup_n-D  NumberOfTableDimensions=1  BreakpointsForDimension1=LoFT.Hydro.waveforces.time + 10  Table=squeeze(LoFT.Hydro.waveforces.force(1,1,:))  InternalRulePriority=Speed  RndMeth=Simplest
  1-D Lookup Table1 : Lookup_n-D  NumberOfTableDimensions=1  BreakpointsForDimension1=LoFT.Hydro.waveforces.time + 10  Table=squeeze(LoFT.Hydro.waveforces.force(1,2,:))  InternalRulePriority=Speed  RndMeth=Simplest
  1-D Lookup Table2 : Lookup_n-D  NumberOfTableDimensions=1  BreakpointsForDimension1=LoFT.Hydro.waveforces.time + 10  Table=squeeze(LoFT.Hydro.waveforces.force(1,3,:))  InternalRulePriority=Speed  RndMeth=Simplest
  Clock1 : Clock
  Clock2 : Clock
  Clock3 : Clock
  Vector Concatenate1 : Concatenate  NumInputs=3
  Out1 : Outport
  wires:
  Vector Concatenate1/1 -> Out1/1
  Clock2/1 -> 1-D Lookup Table1/1
  1-D Lookup Table/1 -> Vector Concatenate1/1
  Clock3/1 -> 1-D Lookup Table2/1
  Clock1/1 -> 1-D Lookup Table/1
  1-D Lookup Table1/1 -> Vector Concatenate1/2
  1-D Lookup Table2/1 -> Vector Concatenate1/3

== system LoFT_Example1/FOWT System/wave series 4 ==
  1-D Lookup Table : Lookup_n-D  NumberOfTableDimensions=1  BreakpointsForDimension1=LoFT.Hydro.waveforces.time+15  Table=squeeze(LoFT.Hydro.waveforces.force(1,1,:))  InternalRulePriority=Speed  RndMeth=Simplest
  1-D Lookup Table1 : Lookup_n-D  NumberOfTableDimensions=1  BreakpointsForDimension1=LoFT.Hydro.waveforces.time+15  Table=squeeze(LoFT.Hydro.waveforces.force(1,2,:))  InternalRulePriority=Speed  RndMeth=Simplest
  1-D Lookup Table2 : Lookup_n-D  NumberOfTableDimensions=1  BreakpointsForDimension1=LoFT.Hydro.waveforces.time+15  Table=squeeze(LoFT.Hydro.waveforces.force(1,3,:))  InternalRulePriority=Speed  RndMeth=Simplest
  Clock1 : Clock
  Clock2 : Clock
  Clock3 : Clock
  Vector Concatenate1 : Concatenate  NumInputs=3
  Out1 : Outport
  wires:
  1-D Lookup Table2/1 -> Vector Concatenate1/3
  1-D Lookup Table1/1 -> Vector Concatenate1/2
  Clock1/1 -> 1-D Lookup Table/1
  Clock3/1 -> 1-D Lookup Table2/1
  1-D Lookup Table/1 -> Vector Concatenate1/1
  Clock2/1 -> 1-D Lookup Table1/1
  Vector Concatenate1/1 -> Out1/1

== system LoFT_Example1/FOWT System/wave series 5 ==
  1-D Lookup Table : Lookup_n-D  NumberOfTableDimensions=1  BreakpointsForDimension1=LoFT.Hydro.waveforces.time+20  Table=squeeze(LoFT.Hydro.waveforces.force(1,1,:))  InternalRulePriority=Speed  RndMeth=Simplest
  1-D Lookup Table1 : Lookup_n-D  NumberOfTableDimensions=1  BreakpointsForDimension1=LoFT.Hydro.waveforces.time+20  Table=squeeze(LoFT.Hydro.waveforces.force(1,2,:))  InternalRulePriority=Speed  RndMeth=Simplest
  1-D Lookup Table2 : Lookup_n-D  NumberOfTableDimensions=1  BreakpointsForDimension1=LoFT.Hydro.waveforces.time+20  Table=squeeze(LoFT.Hydro.waveforces.force(1,3,:))  InternalRulePriority=Speed  RndMeth=Simplest
  Clock1 : Clock
  Clock2 : Clock
  Clock3 : Clock
  Vector Concatenate1 : Concatenate  NumInputs=3
  Out1 : Outport
  wires:
  Vector Concatenate1/1 -> Out1/1
  Clock2/1 -> 1-D Lookup Table1/1
  1-D Lookup Table/1 -> Vector Concatenate1/1
  Clock3/1 -> 1-D Lookup Table2/1
  Clock1/1 -> 1-D Lookup Table/1
  1-D Lookup Table1/1 -> Vector Concatenate1/2
  1-D Lookup Table2/1 -> Vector Concatenate1/3

== system LoFT_Example1/FOWT System/wind series 1 ==
  Clock1 : Clock
  Lookup Table2 : Lookup_n-D  NumberOfTableDimensions=1  BreakpointsForDimension1=Turbwind.WF(1).Time  BreakpointsForDimension2=wind.yDiscr  BreakpointsForDimension3=wind.zDiscr  Table=Turbwind.WF(1).WindVelX  InternalRulePriority=Speed  RndMeth=Simplest
  Out1 : Outport
  wires:
  Lookup Table2/1 -> Out1/1
  Clock1/1 -> Lookup Table2/1

== system LoFT_Example1/FOWT System/wind series 2 ==
  Clock1 : Clock
  Lookup Table2 : Lookup_n-D  NumberOfTableDimensions=1  BreakpointsForDimension1=Turbwind.WF(1).Time  BreakpointsForDimension2=wind.yDiscr  BreakpointsForDimension3=wind.zDiscr  Table=Turbwind.WF(2).WindVelX  InternalRulePriority=Speed  RndMeth=Simplest
  Out1 : Outport
  wires:
  Clock1/1 -> Lookup Table2/1
  Lookup Table2/1 -> Out1/1

== system LoFT_Example1/FOWT System/wind series 3 ==
  Clock1 : Clock
  Lookup Table2 : Lookup_n-D  NumberOfTableDimensions=1  BreakpointsForDimension1=Turbwind.WF(1).Time  BreakpointsForDimension2=wind.yDiscr  BreakpointsForDimension3=wind.zDiscr  Table=Turbwind.WF(3).WindVelX  InternalRulePriority=Speed  RndMeth=Simplest
  Out1 : Outport
  wires:
  Lookup Table2/1 -> Out1/1
  Clock1/1 -> Lookup Table2/1

== system LoFT_Example1/FOWT System/wind series 4 ==
  Clock1 : Clock
  Lookup Table2 : Lookup_n-D  NumberOfTableDimensions=1  BreakpointsForDimension1=Turbwind.WF(1).Time  BreakpointsForDimension2=wind.yDiscr  BreakpointsForDimension3=wind.zDiscr  Table=Turbwind.WF(4).WindVelX  InternalRulePriority=Speed  RndMeth=Simplest
  Out1 : Outport
  wires:
  Clock1/1 -> Lookup Table2/1
  Lookup Table2/1 -> Out1/1

== system LoFT_Example1/FOWT System/wind series 5 ==
  Clock1 : Clock
  Lookup Table2 : Lookup_n-D  NumberOfTableDimensions=1  BreakpointsForDimension1=Turbwind.WF(1).Time  BreakpointsForDimension2=wind.yDiscr  BreakpointsForDimension3=wind.zDiscr  Table=Turbwind.WF(5).WindVelX  InternalRulePriority=Speed  RndMeth=Simplest
  Out1 : Outport
  wires:
  Lookup Table2/1 -> Out1/1
  Clock1/1 -> Lookup Table2/1

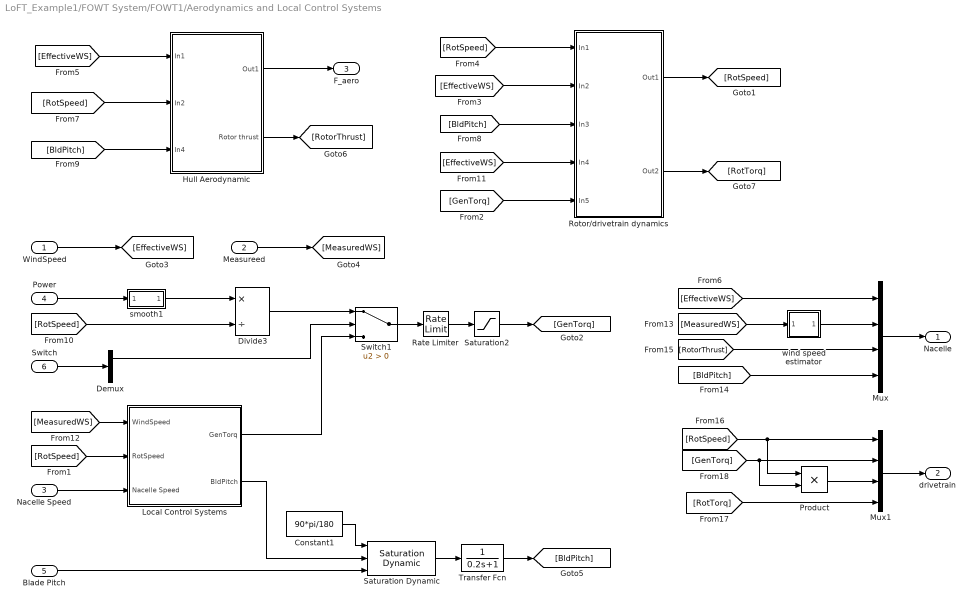
== system LoFT_Example1/FOWT System/FOWT1/Aerodynamics and Local Control Systems ==
  WindSpeed : Inport
  "Measureed " : Inport  Port=2
  Nacelle Speed : Inport  Port=3
  Power : Inport  Port=4
  Blade Pitch : Inport  Port=5
  Switch : Inport  Port=6
  Constant1 : Constant  Value=90*pi/180
  Demux : Demux  Outputs=2
  Divide3 : Product  Inputs=*/
  Hull Aerodynamic : Subsystem
  Local Control Systems : Subsystem
  Mux : Mux
  Mux1 : Mux
  Product : Product
  Rate Limiter : RateLimiter  RisingSlewLimit=Controller.torqueMaxRate  FallingSlewLimit=-Controller.torqueMaxRate  SampleTimeMode=inherited
  Rotor/drivetrain dynamics : Subsystem
  Saturation Dynamic : simulink/Discontinuities/Saturation Dynamic  OutMin=[]  OutMax=[]  OutDataTypeStr=Inherit: Same as second input  OutDataType=fixdt(1, 16)  OutScaling=2^-10  DoSatur=off
  Saturation2 : Saturate  UpperLimit=Controller.torqueMax  LowerLimit=0
  Switch1 : Switch  Criteria=u2 > Threshold  SaturateOnIntegerOverflow=off  InputSameDT=off
  Transfer Fcn : TransferFcn  Denominator=[0.2 1]
  smooth1 : Subsystem
  wind speed estimator : Subsystem
  Nacelle : Outport
  drivetrain : Outport  Port=2
  F_aero : Outport  Port=3
  wires:
  Transfer Fcn/1 -> [BldPitch]
  Mux1/1 -> drivetrain/1
  Mux/1 -> Nacelle/1
  Local Control Systems/2(BldPitch) -> Saturation Dynamic/2
  Saturation Dynamic/1 -> Transfer Fcn/1
  Switch/1 -> Demux/1
  [RotSpeed] -> Divide3/2
  Rate Limiter/1 -> Saturation2/1
  Switch1/1 -> Rate Limiter/1
  Local Control Systems/1(GenTorq) -> Switch1/3
  Divide3/1 -> Switch1/1
  Nacelle Speed/1 -> Local Control Systems/3(Nacelle Speed)
  [RotSpeed] -> Local Control Systems/2(RotSpeed)
  Power/1 -> smooth1/1(In1)
  Blade Pitch/1 -> Saturation Dynamic/3
  Saturation2/1 -> [GenTorq]
  smooth1/1(Out1) -> Divide3/1
  WindSpeed/1 -> [EffectiveWS]
  [EffectiveWS] -> Hull Aerodynamic/1(In1)
  [RotSpeed] -> Hull Aerodynamic/2(In2)
  [BldPitch] -> Hull Aerodynamic/3(In4)
  Hull Aerodynamic/1(Out1) -> F_aero/1
  [RotSpeed] -> Rotor/drivetrain dynamics/1(In1)
  [EffectiveWS] -> Rotor/drivetrain dynamics/2(In2)
  [BldPitch] -> Rotor/drivetrain dynamics/3(In3)
  [EffectiveWS] -> Rotor/drivetrain dynamics/4(In4)
  [GenTorq] -> Rotor/drivetrain dynamics/5(In5)
  Rotor/drivetrain dynamics/1(Out1) -> [RotSpeed]
  [EffectiveWS] -> Mux/1
  [MeasuredWS] -> Local Control Systems/1(WindSpeed)
  "Measureed "/1 -> [MeasuredWS]
  [MeasuredWS] -> wind speed estimator/1(In1)
  wind speed estimator/1(Out1) -> Mux/2
  [BldPitch] -> Mux/4
  Hull Aerodynamic/2(Rotor thrust) -> [RotorThrust]
  [RotorThrust] -> Mux/3
  Demux/1 -> Switch1/2
  [RotSpeed] -> Mux1/1, Product/1
  [GenTorq] -> Mux1/2, Product/2
  Product/1 -> Mux1/3
  Rotor/drivetrain dynamics/2(Out2) -> [RotTorq]
  [RotTorq] -> Mux1/4
  Constant1/1 -> Saturation Dynamic/1

== system LoFT_Example1/FOWT System/FOWT1/Hydrodynamics ==
  Acceleration : Inport
  Speed : Inport  Port=2
  Position : Inport  Port=3
  Wave : Inport  Port=4
  Add : Sum  Inputs=--+
  excitation force : Subsystem
  radiation force : Subsystem
  "viscous force " : Subsystem
  Out1 : Outport
  wires:
  Wave/1 -> excitation force/2(Wave)
  Add/1 -> Out1/1
  excitation force/1(Fext) -> Add/3
  "viscous force "/1(F_vis) -> Add/2
  radiation force/1(F_rad) -> Add/1
  Position/1 -> excitation force/1(position)
  Acceleration/1 -> radiation force/1(velocity)
  Speed/1 -> "viscous force "/1(In1), radiation force/2(In2)

== system LoFT_Example1/FOWT System/FOWT1/Hydrostatics ==
  position : Inport
  Add : Sum
  Add2 : Sum  Inputs=+--
  Assignment : Assignment  DiagnosticForDimensions=Warning  IndexOptions=Index vector (dialog)  Indices=2  OutputSizes=1
  Constant : Constant  Value=Property.masstot-9.7e6
  Constant1 : Constant  Value=Property.volume
  Constant2 : Constant  Value=[0 0 0]
  Constant3 : Constant  Value=4*445087
  Product : Product  Multiplication=Matrix(*)
  "Surge,heave,pitch, Hydro stiffness (3×3)" : Constant  Value=Hydro.hydrostatic
  rho * g : Gain  Gain=1025*9.81
  rho * g1 : Gain  Gain=9.81
  Out1 : Outport
  wires:
  Add2/1 -> Assignment/2
  Add/1 -> Out1/1
  Assignment/1 -> Add/1
  Constant2/1 -> Assignment/1
  rho * g/1 -> Add2/2
  rho * g1/1 -> Add2/1
  Constant/1 -> rho * g1/1
  Product/1 -> Add/2
  Constant1/1 -> rho * g/1
  position/1 -> Product/2
  "Surge,heave,pitch, Hydro stiffness (3×3)"/1 -> Product/1
  Constant3/1 -> Add2/3

== system LoFT_Example1/FOWT System/FOWT1/Measurements ==
  Nacelle : Inport
  drivetrain : Inport  Port=2
  platform : Inport  Port=3
  Bus Creator : BusCreator  Inputs=17
  Demux : Demux  Outputs=9
  Demux1 : Demux
  Demux2 : Demux
  Out1 : Outport
  wires:
  drivetrain/1 -> Demux2/1
  Demux2/4 -> Bus Creator/8  "RotTorq"
  Demux2/3 -> Bus Creator/7  "GenPwr"
  Demux2/2 -> Bus Creator/6  "GenTorq"
  Demux2/1 -> Bus Creator/5  "RotSpeed"
  Demux/1 -> Bus Creator/9  "PtfmSurge"
  Demux/2 -> Bus Creator/10  "PtfmHeave"
  Demux/3 -> Bus Creator/11  "PtfmPitch"
  Demux/4 -> Bus Creator/12  "PtfmTVxi"
  Demux/5 -> Bus Creator/13  "PtfmTVzi"
  Demux/6 -> Bus Creator/14  "PtfmRVyi"
  Demux/7 -> Bus Creator/15  "PtfmTAxi"
  Demux/8 -> Bus Creator/16  "PtfmTAzi"
  Demux/9 -> Bus Creator/17  "PtfmRAyi"
  Demux1/1 -> Bus Creator/1  "WindVelX"
  Demux1/2 -> Bus Creator/2  "WindEst"
  Demux1/3 -> Bus Creator/3  "RotThrust"
  Demux1/4 -> Bus Creator/4  "BldPitch"
  Bus Creator/1 -> Out1/1
  Nacelle/1 -> Demux1/1
  platform/1 -> Demux/1

== system LoFT_Example1/FOWT System/FOWT1/Moorings ==
  position : Inport
  2-D Lookup Table : Lookup_n-D  NumberOfTableDimensions=3  BreakpointsForDimension1=Mooring.X  BreakpointsForDimension2=Mooring.Z  BreakpointsForDimension3=Mooring.RY  Table=Mooring.FX  InternalRulePriority=Speed  RndMeth=Simplest
      settings: InputPortMap=u0,u1,u2
  2-D Lookup Table3 : Lookup_n-D  NumberOfTableDimensions=3  BreakpointsForDimension1=LoFT.Mooring.X  BreakpointsForDimension2=LoFT.Mooring.Z  BreakpointsForDimension3=LoFT.Mooring.RY  Table=LoFT.Mooring.FZ  InternalRulePriority=Speed  RndMeth=Simplest
      settings: InputPortMap=u0,u1,u2
  2-D Lookup Table4 : Lookup_n-D  NumberOfTableDimensions=3  BreakpointsForDimension1=LoFT.Mooring.X  BreakpointsForDimension2=LoFT.Mooring.Z  BreakpointsForDimension3=LoFT.Mooring.RY  Table=LoFT.Mooring.MY  InternalRulePriority=Speed  RndMeth=Simplest
      settings: InputPortMap=u0,u1,u2
  Demux : Demux  Outputs=3
  Demux1 : Demux  Outputs=3
  Demux2 : Demux  Outputs=3
  Vector Concatenate1 : Concatenate  NumInputs=3
  Out1 : Outport
  wires:
  Vector Concatenate1/1 -> Out1/1
  Demux2/2 -> 2-D Lookup Table4/2
  Demux2/1 -> 2-D Lookup Table4/1
  2-D Lookup Table4/1 -> Vector Concatenate1/3
  2-D Lookup Table3/1 -> Vector Concatenate1/2
  Demux1/3 -> 2-D Lookup Table3/3
  Demux/2 -> 2-D Lookup Table/2
  Demux1/1 -> 2-D Lookup Table3/1
  Demux2/3 -> 2-D Lookup Table4/3
  Demux/1 -> 2-D Lookup Table/1
  position/1 -> Demux/1, Demux1/1, Demux2/1
  2-D Lookup Table/1 -> Vector Concatenate1/1
  Demux1/2 -> 2-D Lookup Table3/2
  Demux/3 -> 2-D Lookup Table/3

== system LoFT_Example1/FOWT System/FOWT1/Subsystem1 ==
  In1 : Inport
  In2 : Inport  Port=2
  In3 : Inport  Port=3
  In4 : Inport  Port=4
  In5 : Inport  Port=5
  In6 : Inport  Port=6
  Demux : Demux  Outputs=2
  Demux1 : Demux  Outputs=2
  Demux2 : Demux  Outputs=2
  Mux : Mux  Inputs=9
  Vector Concatenate : Concatenate
  Vector Concatenate1 : Concatenate
  Vector Concatenate2 : Concatenate
  Out4 : Outport
  Out1 : Outport  Port=2
  Out2 : Outport  Port=3
  Out3 : Outport  Port=4
  wires:
  Demux2/2 -> Mux/8
  Demux2/1 -> Mux/7
  Demux1/2 -> Mux/5
  Demux1/1 -> Mux/4
  Demux/2 -> Mux/2
  Demux/1 -> Mux/1
  Mux/1 -> Out4/1
  In6/1 -> Vector Concatenate2/1, Demux2/1
  In2/1 -> Vector Concatenate1/2, Mux/6
  In5/1 -> Vector Concatenate1/1, Demux1/1
  Vector Concatenate/1 -> Out1/1
  Vector Concatenate1/1 -> Out2/1
  Vector Concatenate2/1 -> Out3/1
  In4/1 -> Vector Concatenate/1, Demux/1
  In1/1 -> Vector Concatenate/2, Mux/3
  In3/1 -> Vector Concatenate2/2, Mux/9

== system LoFT_Example1/FOWT System/FOWT1/wind speed(m//s) ==
  Inflow : Inport
  In2 : Inport  Port=2
  Add : Sum
  Demux : Demux  Outputs=3
  Product : Product
  Trigonometric Function : Trigonometry  Operator=cos
  add : Sum  Inputs=+-
  add1 : Sum  Inputs=+-
  hub height : Gain  Gain=145
  Effective : Outport
  Measured : Outport  Port=2
  FB : Outport  Port=3
  wires:
  In2/1 -> Demux/1
  hub height/1 -> Product/1
  Trigonometric Function/1 -> Product/2
  Demux/1 -> Add/1
  Demux/3 -> hub height/1, Trigonometric Function/1
  add/1 -> Effective/1
  add1/1 -> Measured/1
  Product/1 -> Add/2
  Add/1 -> [HubVelocity]
  [HubVelocity] -> add1/2
  [HubVelocity] -> add/2
  [HubVelocity] -> FB/1
  Inflow/1 -> add1/1, add/1

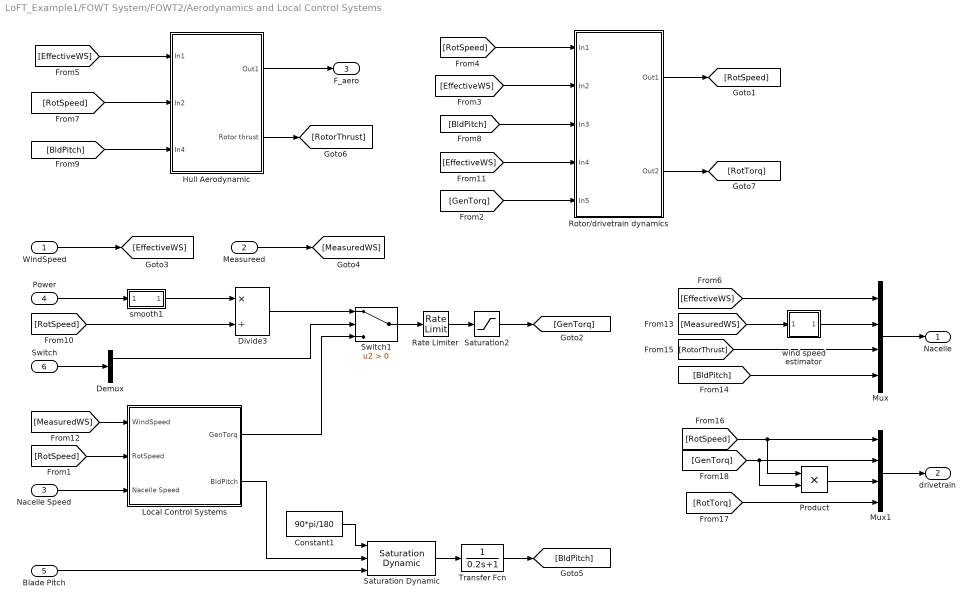
== system LoFT_Example1/FOWT System/FOWT2/Aerodynamics and Local Control Systems ==
  WindSpeed : Inport
  "Measureed " : Inport  Port=2
  Nacelle Speed : Inport  Port=3
  Power : Inport  Port=4
  Blade Pitch : Inport  Port=5
  Switch : Inport  Port=6
  Constant1 : Constant  Value=90*pi/180
  Demux : Demux  Outputs=2
  Divide3 : Product  Inputs=*/
  Hull Aerodynamic : Subsystem
  Local Control Systems : Subsystem
  Mux : Mux
  Mux1 : Mux
  Product : Product
  Rate Limiter : RateLimiter  RisingSlewLimit=Controller.torqueMaxRate  FallingSlewLimit=-Controller.torqueMaxRate  SampleTimeMode=inherited
  Rotor/drivetrain dynamics : Subsystem
  Saturation Dynamic : simulink/Discontinuities/Saturation Dynamic  OutMin=[]  OutMax=[]  OutDataTypeStr=Inherit: Same as second input  OutDataType=fixdt(1, 16)  OutScaling=2^-10  DoSatur=off
  Saturation2 : Saturate  UpperLimit=Controller.torqueMax  LowerLimit=0
  Switch1 : Switch  Criteria=u2 > Threshold  SaturateOnIntegerOverflow=off  InputSameDT=off
  Transfer Fcn : TransferFcn  Denominator=[0.2 1]
  smooth1 : Subsystem
  wind speed estimator : Subsystem
  Nacelle : Outport
  drivetrain : Outport  Port=2
  F_aero : Outport  Port=3
  wires:
  Constant1/1 -> Saturation Dynamic/1
  [RotTorq] -> Mux1/4
  Rotor/drivetrain dynamics/2(Out2) -> [RotTorq]
  Product/1 -> Mux1/3
  [GenTorq] -> Product/2, Mux1/2
  [RotSpeed] -> Product/1, Mux1/1
  Demux/1 -> Switch1/2
  [RotorThrust] -> Mux/3
  Hull Aerodynamic/2(Rotor thrust) -> [RotorThrust]
  [BldPitch] -> Mux/4
  wind speed estimator/1(Out1) -> Mux/2
  [MeasuredWS] -> wind speed estimator/1(In1)
  "Measureed "/1 -> [MeasuredWS]
  [MeasuredWS] -> Local Control Systems/1(WindSpeed)
  [EffectiveWS] -> Mux/1
  Rotor/drivetrain dynamics/1(Out1) -> [RotSpeed]
  [GenTorq] -> Rotor/drivetrain dynamics/5(In5)
  [EffectiveWS] -> Rotor/drivetrain dynamics/4(In4)
  [BldPitch] -> Rotor/drivetrain dynamics/3(In3)
  [EffectiveWS] -> Rotor/drivetrain dynamics/2(In2)
  [RotSpeed] -> Rotor/drivetrain dynamics/1(In1)
  Hull Aerodynamic/1(Out1) -> F_aero/1
  [BldPitch] -> Hull Aerodynamic/3(In4)
  [RotSpeed] -> Hull Aerodynamic/2(In2)
  [EffectiveWS] -> Hull Aerodynamic/1(In1)
  WindSpeed/1 -> [EffectiveWS]
  smooth1/1(Out1) -> Divide3/1
  Saturation2/1 -> [GenTorq]
  Blade Pitch/1 -> Saturation Dynamic/3
  Power/1 -> smooth1/1(In1)
  [RotSpeed] -> Local Control Systems/2(RotSpeed)
  Nacelle Speed/1 -> Local Control Systems/3(Nacelle Speed)
  Divide3/1 -> Switch1/1
  Local Control Systems/1(GenTorq) -> Switch1/3
  Switch1/1 -> Rate Limiter/1
  Rate Limiter/1 -> Saturation2/1
  [RotSpeed] -> Divide3/2
  Switch/1 -> Demux/1
  Saturation Dynamic/1 -> Transfer Fcn/1
  Local Control Systems/2(BldPitch) -> Saturation Dynamic/2
  Mux/1 -> Nacelle/1
  Mux1/1 -> drivetrain/1
  Transfer Fcn/1 -> [BldPitch]

== system LoFT_Example1/FOWT System/FOWT2/Hydrodynamics ==
  Acceleration : Inport
  Speed : Inport  Port=2
  Position : Inport  Port=3
  Wave : Inport  Port=4
  Add : Sum  Inputs=--+
  excitation force : Subsystem
  radiation force : Subsystem
  "viscous force " : Subsystem
  Out1 : Outport
  wires:
  Speed/1 -> radiation force/2(In2), "viscous force "/1(In1)
  Acceleration/1 -> radiation force/1(velocity)
  Position/1 -> excitation force/1(position)
  radiation force/1(F_rad) -> Add/1
  "viscous force "/1(F_vis) -> Add/2
  excitation force/1(Fext) -> Add/3
  Add/1 -> Out1/1
  Wave/1 -> excitation force/2(Wave)

== system LoFT_Example1/FOWT System/FOWT2/Hydrostatics ==
  position : Inport
  Add : Sum
  Add2 : Sum  Inputs=+--
  Assignment : Assignment  DiagnosticForDimensions=Warning  IndexOptions=Index vector (dialog)  Indices=2  OutputSizes=1
  Constant : Constant  Value=Property.masstot-9.7e6
  Constant1 : Constant  Value=Property.volume
  Constant2 : Constant  Value=[0 0 0]
  Constant3 : Constant  Value=4*445087
  Product : Product  Multiplication=Matrix(*)
  "Surge,heave,pitch, Hydro stiffness (3×3)" : Constant  Value=Hydro.hydrostatic
  rho * g : Gain  Gain=1025*9.81
  rho * g1 : Gain  Gain=9.81
  Out1 : Outport
  wires:
  Constant3/1 -> Add2/3
  "Surge,heave,pitch, Hydro stiffness (3×3)"/1 -> Product/1
  position/1 -> Product/2
  Constant1/1 -> rho * g/1
  Product/1 -> Add/2
  Constant/1 -> rho * g1/1
  rho * g1/1 -> Add2/1
  rho * g/1 -> Add2/2
  Constant2/1 -> Assignment/1
  Assignment/1 -> Add/1
  Add/1 -> Out1/1
  Add2/1 -> Assignment/2

== system LoFT_Example1/FOWT System/FOWT2/Measurements ==
  Nacelle : Inport
  drivetrain : Inport  Port=2
  platform : Inport  Port=3
  Bus Creator : BusCreator  Inputs=17
  Demux : Demux  Outputs=9
  Demux1 : Demux
  Demux2 : Demux
  Out1 : Outport
  wires:
  platform/1 -> Demux/1
  Nacelle/1 -> Demux1/1
  Bus Creator/1 -> Out1/1
  Demux1/4 -> Bus Creator/4  "BldPitch"
  Demux1/3 -> Bus Creator/3  "RotThrust"
  Demux1/2 -> Bus Creator/2  "WindEst"
  Demux1/1 -> Bus Creator/1  "WindVelX"
  Demux/9 -> Bus Creator/17  "PtfmRAyi"
  Demux/8 -> Bus Creator/16  "PtfmTAzi"
  Demux/7 -> Bus Creator/15  "PtfmTAxi"
  Demux/6 -> Bus Creator/14  "PtfmRVyi"
  Demux/5 -> Bus Creator/13  "PtfmTVzi"
  Demux/4 -> Bus Creator/12  "PtfmTVxi"
  Demux/3 -> Bus Creator/11  "PtfmPitch"
  Demux/2 -> Bus Creator/10  "PtfmHeave"
  Demux/1 -> Bus Creator/9  "PtfmSurge"
  Demux2/1 -> Bus Creator/5  "RotSpeed"
  Demux2/2 -> Bus Creator/6  "GenTorq"
  Demux2/3 -> Bus Creator/7  "GenPwr"
  Demux2/4 -> Bus Creator/8  "RotTorq"
  drivetrain/1 -> Demux2/1
